simulink model "EnzymeK"  (R2018a)
settings: Solver=VariableStepAuto  StartTime=0.0  StopTime=10.0  RelTol=1e-3
settings Model: Creator=Mahe  LastModifiedBy=Mahe

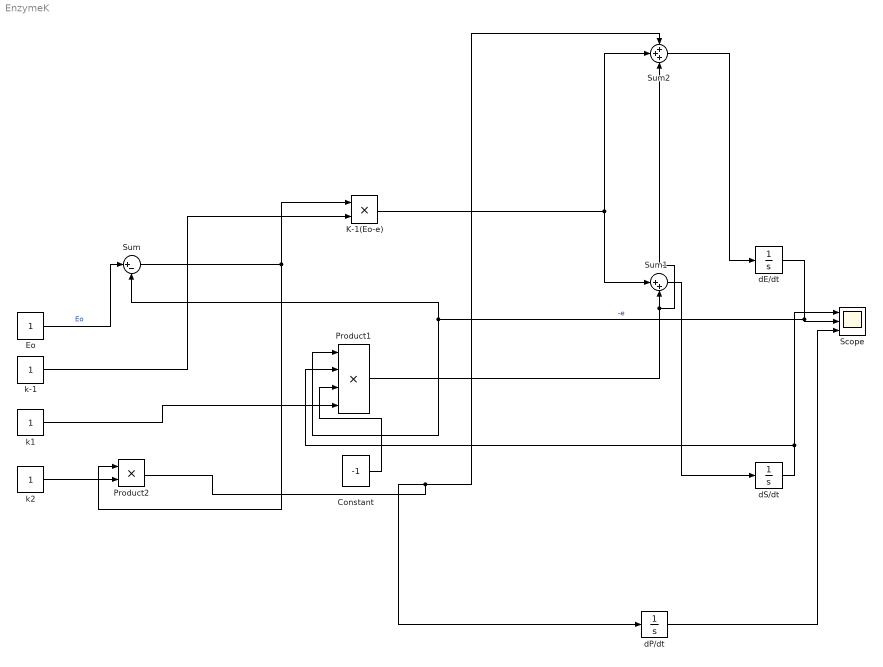
== system EnzymeK ==
  Constant : Constant  Value=-1
  Eo : Constant
  K-1(Eo-e) : Product
  Product1 : Product  Inputs=4
  Product2 : Product
  Scope : Scope  NumInputPorts=3
  Sum : Sum  Inputs=|+-
  Sum1 : Sum  Inputs=|++
  Sum2 : Sum  Inputs=+++
  dE/dt : Integrator  InitialCondition=1
  dP/dt : Integrator
  dS/dt : Integrator  InitialCondition=1
  k-1 : Constant
  k1 : Constant
  k2 : Constant
  wires:
  dS/dt/1 -> Product1/2, Scope/1
  dP/dt/1 -> Scope/3
  dE/dt/1 -> Sum/2, Product1/1, Scope/2  "-e"
  Eo/1 -> Sum/1  "Eo"
  Sum/1 -> K-1(Eo-e)/1, Product2/1
  k-1/1 -> K-1(Eo-e)/2
  k1/1 -> Product1/4
  Constant/1 -> Product1/3
  K-1(Eo-e)/1 -> Sum1/1, Sum2/2
  Product1/1 -> Sum2/3, Sum1/2
  Sum1/1 -> dS/dt/1
  k2/1 -> Product2/2
  Product2/1 -> dP/dt/1, Sum2/1
  Sum2/1 -> dE/dt/1
